simulink model "actual_01_physical_system"  (R2024b)
settings: Solver=VariableStepAuto  StartTime=0.0  StopTime=10.0  RelTol=1e-3
settings Model: Creator=santi  LastModifiedBy=santi

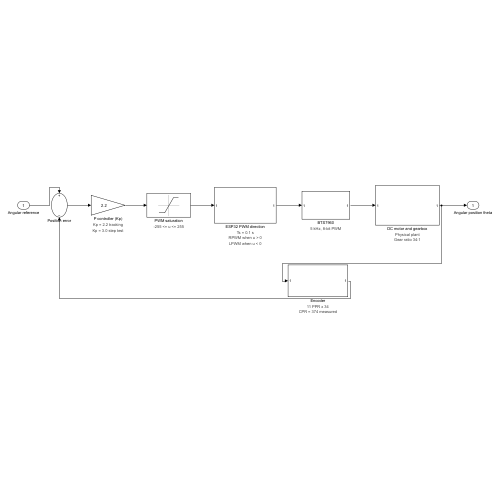
[thumbnail: Simulink's stored preview of the top-level diagram]
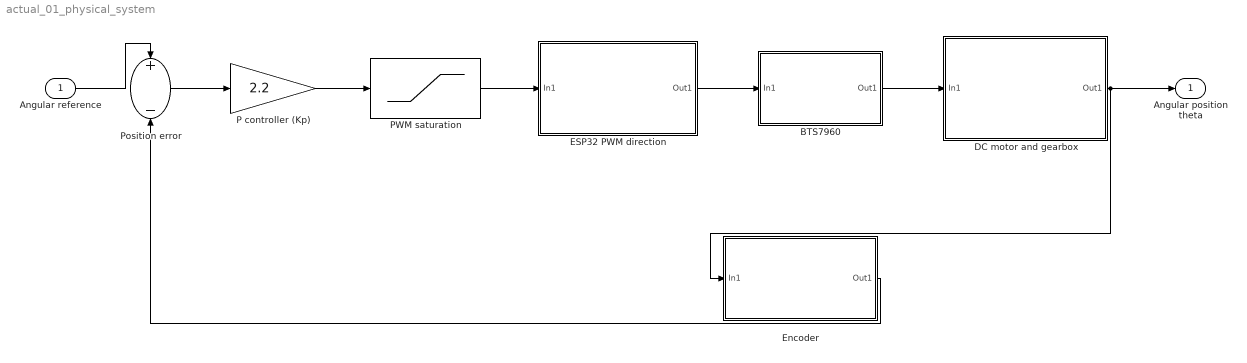
== system actual_01_physical_system ==
  Angular reference : Inport
  BTS7960 : Subsystem
      settings: AttributesFormatString=5 kHz, 8-bit PWM
  DC motor and gearbox : Subsystem
      settings: AttributesFormatString=|
      | Physical plant
      | Gear ratio 34:1
  ESP32 PWM direction : Subsystem
      settings: AttributesFormatString=|
      | Ts = 0.1 s
      | RPWM when u > 0
      | LPWM when u < 0
  Encoder : Subsystem
      settings: AttributesFormatString=|
      | 11 PPR x 34
      | CPR = 374 measured
  P controller (Kp) : Gain  Gain=2.2
      settings: AttributesFormatString=|
      | Kp = 2.2 tracking
      | Kp = 3.0 step test
  PWM saturation : Saturate  UpperLimit=255  LowerLimit=-255
      settings: AttributesFormatString=-255 <= u <= 255
  Position error : Sum  Inputs=+-
  Angular position theta : Outport
  wires:
  Angular reference/1 -> Position error/1
  Position error/1 -> P controller (Kp)/1
  P controller (Kp)/1 -> PWM saturation/1
  PWM saturation/1 -> ESP32 PWM direction/1(In1)
  ESP32 PWM direction/1(Out1) -> BTS7960/1(In1)
  BTS7960/1(Out1) -> DC motor and gearbox/1(In1)
  DC motor and gearbox/1(Out1) -> Angular position theta/1, Encoder/1(In1)
  Encoder/1(Out1) -> Position error/2

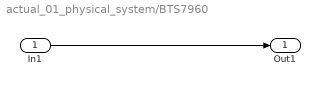
== system actual_01_physical_system/BTS7960 ==
  In1 : Inport
  Out1 : Outport
  wires:
  In1/1 -> Out1/1

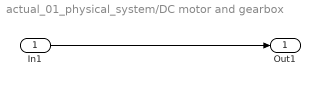
== system actual_01_physical_system/DC motor and gearbox ==
  In1 : Inport
  Out1 : Outport
  wires:
  In1/1 -> Out1/1

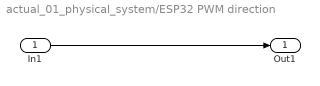
== system actual_01_physical_system/ESP32 PWM direction ==
  In1 : Inport
  Out1 : Outport
  wires:
  In1/1 -> Out1/1

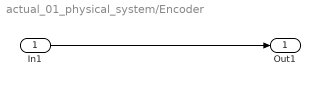
== system actual_01_physical_system/Encoder ==
  In1 : Inport
  Out1 : Outport
  wires:
  In1/1 -> Out1/1
